simulink library "stringblocks"  (Simulink 6.0)
settings: Solver=ode45  SolverMode=SingleTasking  StartTime=0.0  StopTime=10.0  RelTol=1e-3
libraries: target_mpc555 x1, simulink3 x1
settings Model: Creator=The MathWorks Inc.  LastModifiedBy=batserve  ExtModeAutoUpdateStatusClock=off
settings OptimizationCC: BooleanDataType=off
settings DebuggingCC: CheckExecutionContextPreStartOutputMsg=on  CheckExecutionContextRuntimeOutputMsg=on  SolverPrmCheckMsg=none
settings HardwareCC: TargetUnknown=on

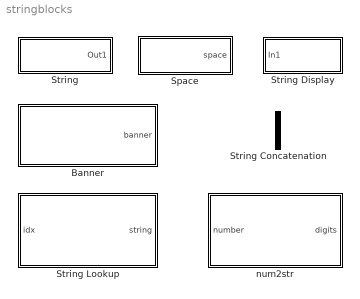
== system stringblocks ==
  Banner : Subsystem  PropExecContextAcrossSSBoundary=on  mask(Banner){banner=Banner text, t=1, banner_width=10}
      mask prompts: banner "String"; t "Sample Time"; banner_width "Visible Banner Width"
      mask help:
      | The output of this block is a sliding window over the banner string.
      |
      | The output is standard ASCII codes output as a wide uint8 signal.
      mask Display:
      | text(0.5,0.8,[ num2str(banner_width) 'char wide banner' ],'horizontalalignment','center')
      | disp(banner)
      | plot([0.25 0.75 0.75 0.25 0.25],[0.3 0.3 0.7 0.7 0.3])
      | plot([0.25 0.5],[0.1 0.1]);
      | plot([0.4 0.5 0.4 0.4],[0.175 0.1 0.025 0.175])
  Space : Subsystem  PropExecContextAcrossSSBoundary=on
      mask Type: Single White Space
      mask Description: When you mux strings together you can insert this block to make sure there is whitespace between the strings.
      mask Display: disp('''  ''');
  String : Subsystem  PropExecContextAcrossSSBoundary=on  mask(String Output){S=String text}
      mask prompts: S "String"
      mask help: Represent the string in standard ASCII code as a wide uint8 signal.
      mask init:
      | u = uint8(S);
      mask Display: disp(S)
  String Concatenation : Mux  Inputs=2
  String Display : Subsystem  PropExecContextAcrossSSBoundary=on  mask(String Display){S=}
      mask help: Displays a vector of characters as a string on the block. The input should be a wide vector. Each element in the vector should be the numerical ASCII code for that character.
      mask init:
      | block=gcb;
      mask Display: disp(S)
  String Lookup : Subsystem  PropExecContextAcrossSSBoundary=on  mask(String Lookup){S={'a'; 'b'; 'c'}}
      mask prompts: S "Strings"
      mask help:
      | Specify a cell array of strings as a lookup table.
      |
      | The input to the block is base zero addressing so the first string will be output if the input is 0. The output is standard ASCII code and will be a wide uint8 vector as wide as the largest string in the cell array set.
      mask init:
      | SS = S;
      | SS = [ sprintf('%s\\n',S{1:end-1}) S{end} ];
      | S = uint8(strvcat(S{:}))';
      | 
      | if size(S,2)<=1
      |    error('You must have at least two strings for the lookup table');
      | end
      mask Display:
      | text(0.1,0.9,'STRING LOOKUP :');
      | text(0.2,0.4,SS)
      | 
      | plot([0.15 0.15],[0 0.8]);
      | plot([0.15 0.5],[0 0])
      | plot([0.15 0.5],[0.8 0.8])
  num2str : Subsystem  TreatAsAtomicUnit=on  PropExecContextAcrossSSBoundary=on  mask(Num2Str){N=6, S=1, O=0, B=10}
      mask prompts: N "Number of digits"; S "Scaling"; O "Offset"; B "Base"
      mask help:
      | Converts an input number to a string output.
      |
      | Given the scaling and offset and the number of digits to output a string is represented in standard ASCII codes as a wide uint8 signal line.
      mask init:
      | if B <=0 | B >10
      |    error('Base must be between 1 and 10');
      | end
      mask Help: Converts an input number to a string output given the scaling and offset and the number of digits to output. The string is output in standard ASCII codes as a wide uint8 signal line.
      mask Display: text(0.1,0.5,sprintf('Number to String\\n   digits      %d\\n   scaling   %g\\n   offset      %g',N,S,O))

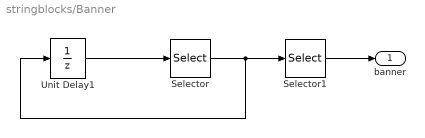
== system stringblocks/Banner ==
  Selector : Selector  Elements=[2:length(banner) 1 ]  InputPortWidth=length(banner)
  Selector1 : Selector  Elements=[1:banner_width]
  Unit Delay1 : UnitDelay  X0=uint8(banner)  SampleTime=t
  banner : Outport
  wires:
  Selector1/1 -> banner/1
  Unit Delay1/1 -> Selector/1
  Selector/1 -> Selector1/1, Unit Delay1/1

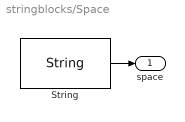
== system stringblocks/Space ==
  String : target_mpc555/String Operations/String  S=""
  space : Outport
  wires:
  String/1 -> space/1

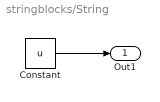
== system stringblocks/String ==
  Constant : Constant  Value=u
  Out1 : Outport
  wires:
  Constant/1 -> Out1/1

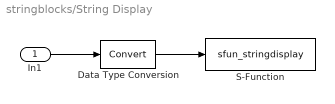
== system stringblocks/String Display ==
  In1 : Inport  Port=1  LatchInput=off
  Data Type Conversion : DataTypeConversion  SaturateOnIntegerOverflow=on  RndMeth=Zero
  S-Function : S-Function  FunctionName=sfun_stringdisplay  Parameters=block  mask{block=block, S=1}
      mask Display: disp(S)
  wires:
  Data Type Conversion/1 -> S-Function/1
  In1/1 -> Data Type Conversion/1

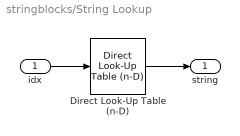
== system stringblocks/String Lookup ==
  idx : Inport  Port=1  LatchInput=off
  Direct Look-Up Table (n-D) : simulink3/Functions & Tables/Direct Look-Up Table (n-D)  maskTabDims=2  explicitNumDims=1  outDims=Column  tabIsInput=off  mxTable=S  clipFlag=Warning
  string : Outport
  wires:
  Direct Look-Up Table (n-D)/1 -> string/1
  idx/1 -> Direct Look-Up Table (n-D)/1

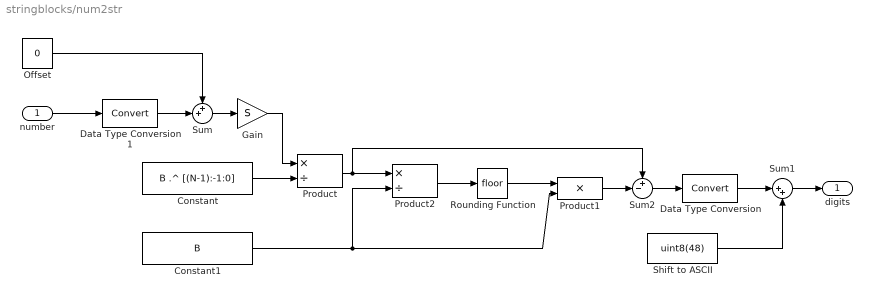
== system stringblocks/num2str ==
  number : Inport  Port=1  LatchInput=off
  Constant : Constant  Value=B .^ [(N-1):-1:0]
  Constant1 : Constant  Value=B
  Data Type Conversion : DataTypeConversion  RndMeth=Zero
  Data Type Conversion1 : DataTypeConversion  RndMeth=Zero
  Gain : Gain  Gain=S  SaturateOnIntegerOverflow=on
  Offset : Constant  Value=0
  Product : Product  Inputs=*/  SaturateOnIntegerOverflow=on  RndMeth=Zero  InputSameDT=on
  Product1 : Product  Inputs=**  SaturateOnIntegerOverflow=on  RndMeth=Zero  InputSameDT=on
  Product2 : Product  Inputs=*/  SaturateOnIntegerOverflow=on  RndMeth=Zero  InputSameDT=on
  Rounding Function : Rounding
  Shift to ASCII : Constant  Value=uint8(48)
  Sum : Sum  Inputs=++|  SaturateOnIntegerOverflow=on  InputSameDT=on
  Sum1 : Sum  Inputs=|++  InputSameDT=on
  Sum2 : Sum  Inputs=+-|  InputSameDT=on
  digits : Outport
  wires:
  Data Type Conversion1/1 -> Sum/2
  Offset/1 -> Sum/1
  Data Type Conversion/1 -> Sum1/1
  Sum2/1 -> Data Type Conversion/1
  Product2/1 -> Rounding Function/1
  Product/1 -> Sum2/1, Product2/1
  Rounding Function/1 -> Product1/1
  Shift to ASCII/1 -> Sum1/2
  Sum1/1 -> digits/1
  Gain/1 -> Product/1
  Sum/1 -> Gain/1
  number/1 -> Data Type Conversion1/1
  Constant/1 -> Product/2
  Constant1/1 -> Product2/2, Product1/2
  Product1/1 -> Sum2/2
